simulink model "q1w8"  (R2014b)
settings: Solver=ode23  StartTime=0.0  StopTime=10.0  RelTol=1e-3
undefined symbols (not defined in the file or in its folder): k
settings Model: Creator=Student  LastModifiedBy=Student

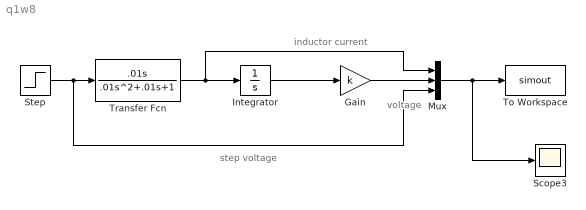
== system q1w8 ==
  note: voltage
  note: inductor current
  note: step voltage
  Gain : Gain  Gain=k
  Integrator : Integrator
  Mux : Mux  Inputs=3
  Scope3 : Scope
      settings: ShowLegends=on  SaveName=ScopeData3
  Step : Step  After=10  SampleTime=0
  To Workspace : ToWorkspace  VariableName=simout  SaveFormat=Timeseries  SampleTime=-1
  Transfer Fcn : TransferFcn  Numerator=[.01 0]  Denominator=[.01 .01 1]
  wires:
  Transfer Fcn/1 -> Mux/1, Integrator/1
  Integrator/1 -> Gain/1
  Gain/1 -> Mux/2
  Mux/1 -> Scope3/1, To Workspace/1
  Step/1 -> Mux/3, Transfer Fcn/1
